simulink model "PiezoDrucksensore_Model"  (R2015b)
settings: Solver=VariableStepAuto  StartTime=0.0  StopTime=10.0  RelTol=1e-3
values from neighbouring files (symbols this model uses):
  C = 1E-6    (= 1e-06)    [Piezo_TF_Model.m]
  CD = 10E-9    (= 1e-08)    [Piezo_TF_Model.m]
  R = 100E+6    (= 100000000)    [Piezo_TF_Model.m]
  RD = 1E+9    (= 1000000000)    [Piezo_TF_Model.m]
  v0 = 100E+3    (= 100000)    [Piezo_TF_Model.m]
  w0 = 10    [Piezo_TF_Model.m]
settings Model: Creator=lukaskiechle  LastModifiedBy=lukaskiechle

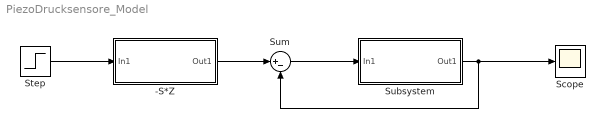
== system PiezoDrucksensore_Model ==
  -S*Z : Subsystem
  Scope : Scope
  Step : Step  SampleTime=0
  Subsystem : Subsystem
  Sum : Sum  Inputs=|+-
  wires:
  Step/1 -> -S*Z/1(In1)
  -S*Z/1(Out1) -> Sum/1
  Sum/1 -> Subsystem/1(In1)
  Subsystem/1(Out1) -> Sum/2, Scope/1

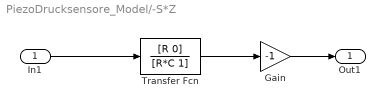
== system PiezoDrucksensore_Model/-S*Z ==
  In1 : Inport
  Gain : Gain  Gain=-1
  Transfer Fcn : TransferFcn  Numerator=[R 0]  Denominator=[R*C 1]
  Out1 : Outport
  wires:
  In1/1 -> Transfer Fcn/1
  Gain/1 -> Out1/1
  Transfer Fcn/1 -> Gain/1

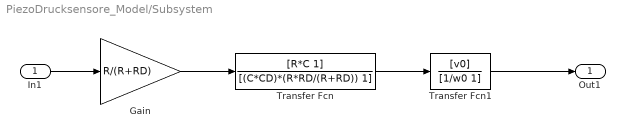
== system PiezoDrucksensore_Model/Subsystem ==
  In1 : Inport
  Gain : Gain  Gain=R/(R+RD)
  Transfer Fcn : TransferFcn  Numerator=[R*C 1]  Denominator=[(C*CD)*(R*RD/(R+RD)) 1]
  Transfer Fcn1 : TransferFcn  Numerator=[v0]  Denominator=[1/w0 1]
  Out1 : Outport
  wires:
  Transfer Fcn/1 -> Transfer Fcn1/1
  Transfer Fcn1/1 -> Out1/1
  Gain/1 -> Transfer Fcn/1
  In1/1 -> Gain/1
